simulink model "FD_2doF"  (R2019b)
settings: Solver=VariableStepAuto  StartTime=0.0  StopTime=10.0  RelTol=1e-3
InitFcn:
  | load("parameters.mat");
  | load("Coefficients.mat");
undefined symbols (not defined in the file): Dm, Dt, g, Jp, Jy, k_pitch, k_py, k_yaw, k_yp, Mb, w_neg, w_pos
libraries: cstblocks x3
settings Model: Creator=laptop  LastModifiedBy=lbend

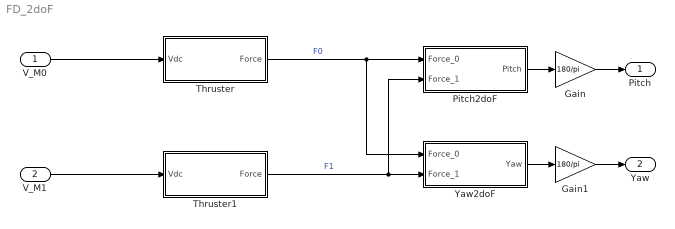
== system FD_2doF ==
  "V_M0 " : Inport
  "V_M1 " : Inport  Port=2
  Gain : Gain  Gain=180/pi
  Gain1 : Gain  Gain=180/pi
  Pitch2doF : Subsystem
  Thruster : Subsystem
  Thruster1 : Subsystem
  Yaw2doF : Subsystem
  Pitch : Outport
  "Yaw " : Outport  Port=2
  wires:
  "V_M1 "/1 -> Thruster1/1(Vdc)
  Thruster/1(Force) -> Yaw2doF/1(Force_0), Pitch2doF/1(Force_0)  "F0"
  "V_M0 "/1 -> Thruster/1(Vdc)
  Thruster1/1(Force) -> Pitch2doF/2(Force_1), Yaw2doF/2(Force_1)  "F1"
  Pitch2doF/1(Pitch) -> Gain/1
  Yaw2doF/1(Yaw) -> Gain1/1
  Gain/1 -> Pitch/1
  Gain1/1 -> "Yaw "/1

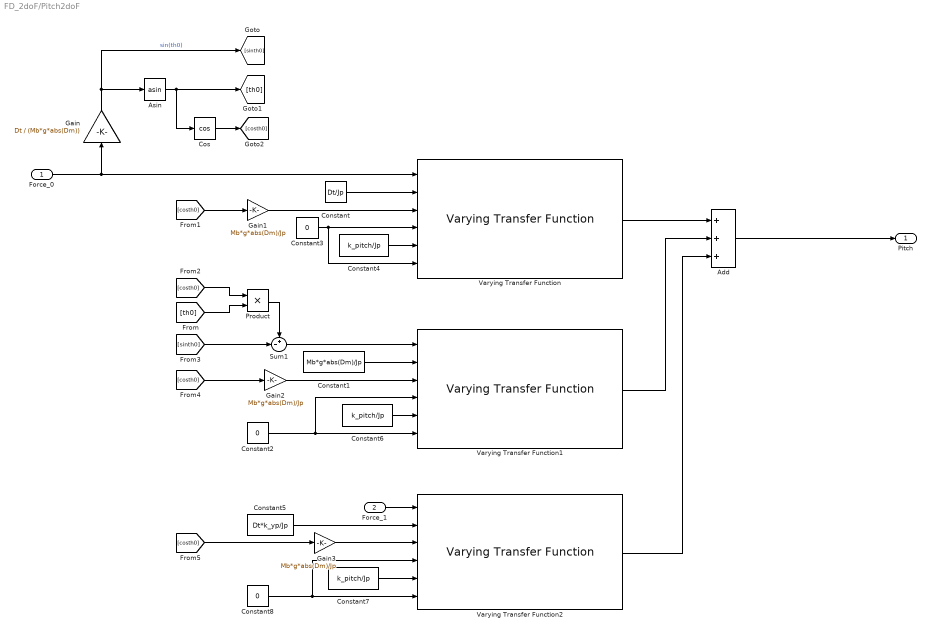
== system FD_2doF/Pitch2doF ==
  Force_0 : Inport
  Force_1 : Inport  Port=2
  Add : Sum  Inputs=+++
  Asin : Trigonometry  Operator=asin
  Constant : Constant  Value=Dt/Jp  SampleTime=0
  Constant1 : Constant  Value=Mb*g*abs(Dm)/Jp  SampleTime=0
  Constant2 : Constant  Value=0  SampleTime=0
  Constant3 : Constant  Value=0  SampleTime=0
  Constant4 : Constant  Value=k_pitch/Jp  SampleTime=0
  Constant5 : Constant  Value=Dt*k_yp/Jp  SampleTime=0
  Constant6 : Constant  Value=k_pitch/Jp  SampleTime=0
  Constant7 : Constant  Value=k_pitch/Jp  SampleTime=0
  Constant8 : Constant  Value=0  SampleTime=0
  Cos : Trigonometry  Operator=cos
  Gain : Gain  Gain=Dt / (Mb*g*abs(Dm))
  Gain1 : Gain  Gain=Mb*g*abs(Dm)/Jp
  Gain2 : Gain  Gain=Mb*g*abs(Dm)/Jp
  Gain3 : Gain  Gain=Mb*g*abs(Dm)/Jp
  Product : Product
  Sum1 : Sum  Inputs=+-|
  Varying Transfer Function : cstblocks/Linear Parameter Varying/Varying Transfer Function  N=2
      settings: SourceProductName=Control System Toolbox
  Varying Transfer Function1 : cstblocks/Linear Parameter Varying/Varying Transfer Function  N=2
      settings: SourceProductName=Control System Toolbox
  Varying Transfer Function2 : cstblocks/Linear Parameter Varying/Varying Transfer Function  N=2
      settings: SourceProductName=Control System Toolbox
  Pitch : Outport
  wires:
  Force_0/1 -> Varying Transfer Function/1, Gain/1
  Constant8/1 -> Varying Transfer Function2/6, Varying Transfer Function2/4
  [costh0] -> Gain2/1
  Constant1/1 -> Varying Transfer Function1/2
  Cos/1 -> [costh0]
  Product/1 -> Sum1/1
  [th0] -> Product/2
  Gain2/1 -> Varying Transfer Function1/3
  Constant3/1 -> Varying Transfer Function/4, Varying Transfer Function/6
  Constant4/1 -> Varying Transfer Function/5
  Constant6/1 -> Varying Transfer Function1/5
  Constant7/1 -> Varying Transfer Function2/5
  [sinth0] -> Sum1/2
  [costh0] -> Gain3/1
  Gain3/1 -> Varying Transfer Function2/3
  [costh0] -> Gain1/1
  Gain1/1 -> Varying Transfer Function/3
  Varying Transfer Function1/1 -> Add/2
  Gain/1 -> Asin/1, [sinth0]  "sin(th0)"
  Sum1/1 -> Varying Transfer Function1/1
  Constant2/1 -> Varying Transfer Function1/6, Varying Transfer Function1/4
  Constant5/1 -> Varying Transfer Function2/2
  Constant/1 -> Varying Transfer Function/2
  Asin/1 -> [th0], Cos/1
  Force_1/1 -> Varying Transfer Function2/1
  Varying Transfer Function/1 -> Add/1
  Varying Transfer Function2/1 -> Add/3
  Add/1 -> Pitch/1
  [costh0] -> Product/1

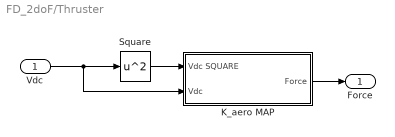
== system FD_2doF/Thruster ==
  Vdc : Inport
  K_aero MAP : Subsystem
  Square : Math  Operator=square  SignedPower=off  SaturateOnIntegerOverflow=on
  Force : Outport
  wires:
  Vdc/1 -> K_aero MAP/2(Vdc), Square/1
  Square/1 -> K_aero MAP/1(Vdc SQUARE)
  K_aero MAP/1(Force) -> Force/1

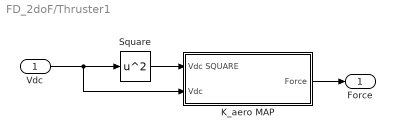
== system FD_2doF/Thruster1 ==
  Vdc : Inport
  K_aero MAP : Subsystem
  Square : Math  Operator=square  SignedPower=off  SaturateOnIntegerOverflow=on
  Force : Outport
  wires:
  Vdc/1 -> K_aero MAP/2(Vdc), Square/1
  Square/1 -> K_aero MAP/1(Vdc SQUARE)
  K_aero MAP/1(Force) -> Force/1

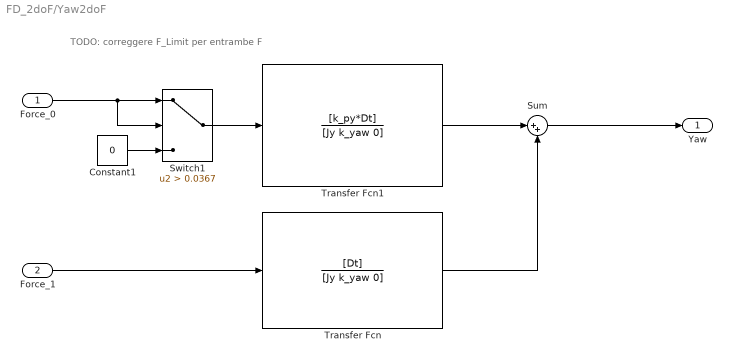
== system FD_2doF/Yaw2doF ==
  note: TODO: correggere F_Limit
      | per entrambe F
  Force_0 : Inport
  Force_1 : Inport  Port=2
  Constant1 : Constant  Value=0
  Sum : Sum  Inputs=|++
  Switch1 : Switch  Criteria=u2 > Threshold  Threshold=0.0367
  Transfer Fcn : TransferFcn  Numerator=[Dt]  Denominator=[Jy k_yaw 0]
  Transfer Fcn1 : TransferFcn  Numerator=[k_py*Dt]  Denominator=[Jy k_yaw 0]
  Yaw : Outport
  wires:
  Transfer Fcn/1 -> Sum/2
  Sum/1 -> Yaw/1
  Switch1/1 -> Transfer Fcn1/1
  Constant1/1 -> Switch1/3
  Force_1/1 -> Transfer Fcn/1
  Force_0/1 -> Switch1/2, Switch1/1
  Transfer Fcn1/1 -> Sum/1

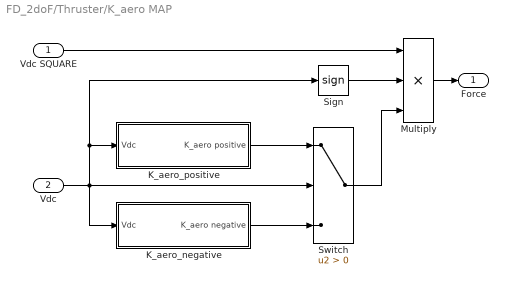
== system FD_2doF/Thruster/K_aero MAP ==
  Vdc SQUARE : Inport
  Vdc : Inport  Port=2
  K_aero_negative : Subsystem
  K_aero_positive : Subsystem
  "Multiply " : Product  Inputs=***
  Sign : Signum
  Switch : Switch  Criteria=u2 > Threshold
  Force : Outport
  wires:
  Vdc SQUARE/1 -> "Multiply "/1
  "Multiply "/1 -> Force/1
  Vdc/1 -> K_aero_negative/1(Vdc), Switch/2, Sign/1, K_aero_positive/1(Vdc)
  K_aero_positive/1(K_aero positive) -> Switch/1
  K_aero_negative/1(K_aero negative) -> Switch/3
  Switch/1 -> "Multiply "/3
  Sign/1 -> "Multiply "/2

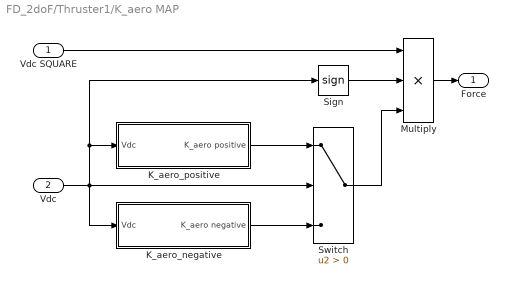
== system FD_2doF/Thruster1/K_aero MAP ==
  Vdc SQUARE : Inport
  Vdc : Inport  Port=2
  K_aero_negative : Subsystem
  K_aero_positive : Subsystem
  "Multiply " : Product  Inputs=***
  Sign : Signum
  Switch : Switch  Criteria=u2 > Threshold
  Force : Outport
  wires:
  Vdc SQUARE/1 -> "Multiply "/1
  "Multiply "/1 -> Force/1
  Vdc/1 -> K_aero_negative/1(Vdc), Switch/2, Sign/1, K_aero_positive/1(Vdc)
  K_aero_positive/1(K_aero positive) -> Switch/1
  K_aero_negative/1(K_aero negative) -> Switch/3
  Switch/1 -> "Multiply "/3
  Sign/1 -> "Multiply "/2

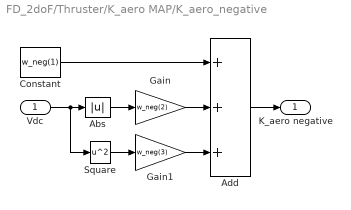
== system FD_2doF/Thruster/K_aero MAP/K_aero_negative ==
  Vdc : Inport
  Abs : Abs
  Add : Sum  Inputs=+++
  Constant : Constant  Value=w_neg(1)  SampleTime=0
  Gain : Gain  Gain=w_neg(2)
  Gain1 : Gain  Gain=w_neg(3)
  Square : Math  Operator=square  SignedPower=off  SaturateOnIntegerOverflow=on
  K_aero negative : Outport
  wires:
  Gain1/1 -> Add/3
  Add/1 -> K_aero negative/1
  Constant/1 -> Add/1
  Gain/1 -> Add/2
  Square/1 -> Gain1/1
  Abs/1 -> Gain/1
  Vdc/1 -> Square/1, Abs/1

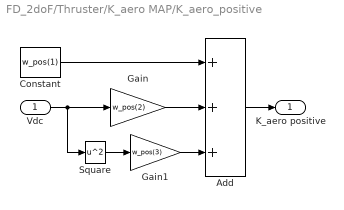
== system FD_2doF/Thruster/K_aero MAP/K_aero_positive ==
  Vdc : Inport
  Add : Sum  Inputs=+++
  Constant : Constant  Value=w_pos(1)  SampleTime=0
  Gain : Gain  Gain=w_pos(2)
  Gain1 : Gain  Gain=w_pos(3)
  Square : Math  Operator=square  SignedPower=off  SaturateOnIntegerOverflow=on
  K_aero positive : Outport
  wires:
  Constant/1 -> Add/1
  Vdc/1 -> Square/1, Gain/1
  Add/1 -> K_aero positive/1
  Gain/1 -> Add/2
  Square/1 -> Gain1/1
  Gain1/1 -> Add/3

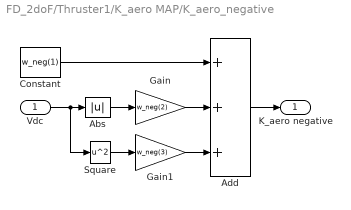
== system FD_2doF/Thruster1/K_aero MAP/K_aero_negative ==
  Vdc : Inport
  Abs : Abs
  Add : Sum  Inputs=+++
  Constant : Constant  Value=w_neg(1)  SampleTime=0
  Gain : Gain  Gain=w_neg(2)
  Gain1 : Gain  Gain=w_neg(3)
  Square : Math  Operator=square  SignedPower=off  SaturateOnIntegerOverflow=on
  K_aero negative : Outport
  wires:
  Gain1/1 -> Add/3
  Add/1 -> K_aero negative/1
  Constant/1 -> Add/1
  Gain/1 -> Add/2
  Square/1 -> Gain1/1
  Abs/1 -> Gain/1
  Vdc/1 -> Square/1, Abs/1

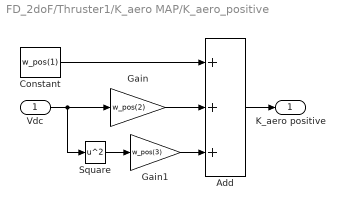
== system FD_2doF/Thruster1/K_aero MAP/K_aero_positive ==
  Vdc : Inport
  Add : Sum  Inputs=+++
  Constant : Constant  Value=w_pos(1)  SampleTime=0
  Gain : Gain  Gain=w_pos(2)
  Gain1 : Gain  Gain=w_pos(3)
  Square : Math  Operator=square  SignedPower=off  SaturateOnIntegerOverflow=on
  K_aero positive : Outport
  wires:
  Constant/1 -> Add/1
  Vdc/1 -> Square/1, Gain/1
  Add/1 -> K_aero positive/1
  Gain/1 -> Add/2
  Square/1 -> Gain1/1
  Gain1/1 -> Add/3
